simulink model "Projectsim"  (R2024a)
settings: Solver=VariableStepAuto  StartTime=0.0  StopTime=10.0  RelTol=1e-3
libraries: spsDiodeLib x8, spsCurrentMeasurementLib x4, spsGtoLib x4, spsSeriesRLCBranchLib x4, spsVoltageMeasurementLib x4, spsDCVoltageSourceLib x1, spsLinearTransformerLib x1, sps_lib x1
settings Model: Creator=yashp  LastModifiedBy=yashp

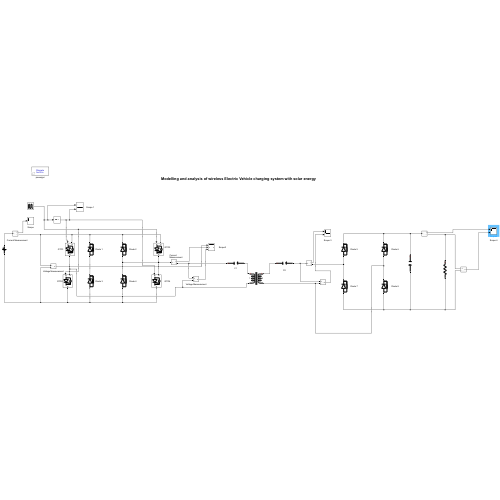
[thumbnail: Simulink's stored preview of the top-level diagram]
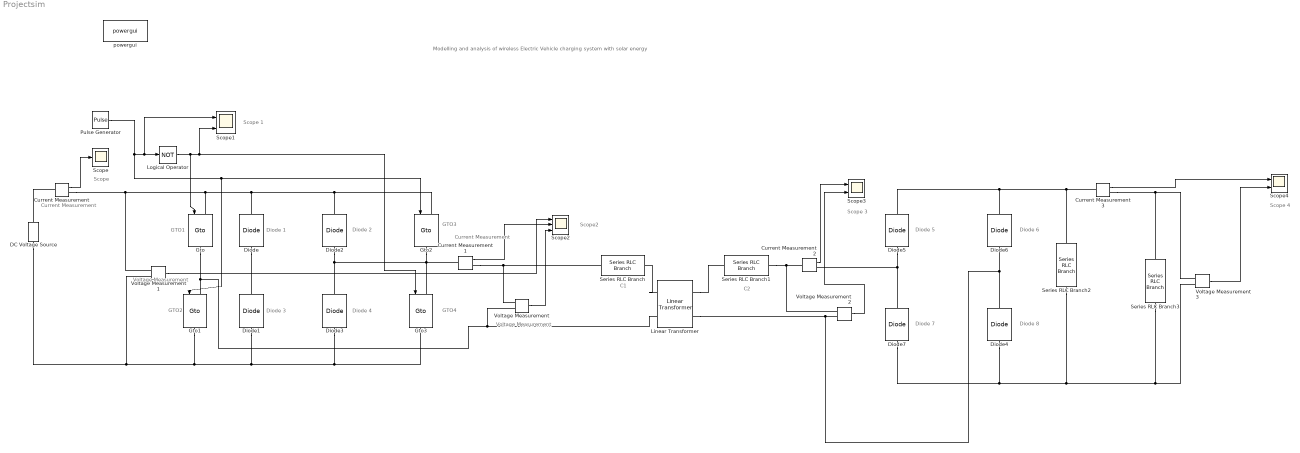
== system Projectsim ==
  note: Diode 8
  note: Diode 7
  note: Diode 6
  note: Diode 5
  note: C2
  note: C1
  note: Scope 4
  note: Scope 3
  note: Scope2
  note: Voltage Measurement
  note: Current
      | Measurement
  note: Scope 1
  note: Scope
  note: Voltage Measurement
  note: Current Measurement
  note: Diode 4
  note: Diode 3
  note: Diode 2
  note: Diode 1
  note: GTO4
  note: GTO3
  note: GTO2
  note: GTO1
  note: Modelling and analysis of wireless Electric Vehicle charging system with solar energy
  Current Measurement{,1..3} (4 alike) : spsCurrentMeasurementLib/Current Measurement  PhasorSimulation=off  OutputType=Complex  PSBequivalent=0
  DC Voltage Source : spsDCVoltageSourceLib/DC Voltage Source  Amplitude=228  Measurements=None
  Diode{,1..7} (8 alike) : spsDiodeLib/Diode  Ron=0.001  Lon=0  Vf=0.8  IC=0  UseSnubber=0  Rs=500  Cs=250e-9  Measurements=off
  Gto{,1..3} (4 alike) : spsGtoLib/Gto  Ron=0.001  Lon=0  Vf=1  Tf=10e-6  Tt=20e-6  IC=0  Rs=1e5  Cs=inf  Measurements=off
      settings: LibrarySourceBlock=sps_lib/Power Electronics/Gto
  Linear Transformer : spsLinearTransformerLib/Linear Transformer  UNITS=pu  NominalPower=[ 250e6 60 ]  winding1="[ 735e3  0.002  0.08 ]"  winding2="[ 315e3  0.002  0.08 ]"  ThreeWindings=off  winding3=[ 315e3 0.002 0.08 ]  RmLm=[ 500 500 ]  Measurements=None  DataType=off
  Logical Operator : Logic  Operator=NOT  AllPortsSameDT=off  OutDataTypeStr=boolean
  Pulse Generator : DiscretePulseGenerator  PulseType=Time based  Period=2.4096e-05  PulseWidth=50
  Scope : Scope
  Scope1 : Scope  NumInputPorts=2
  Scope2 : Scope  NumInputPorts=3
  Scope3 : Scope  NumInputPorts=2
  Scope4 : Scope  NumInputPorts=2
  Series RLC Branch : spsSeriesRLCBranchLib/Series RLC Branch  LConnTagsString=__new0  RConnTagsString=__new0  BranchType=C  Resistance=1  Inductance=1e-3  SetiL0=off  InitialCurrent=0  Capacitance=1e-6  Setx0=off  InitialVoltage=0  Measurements=None
  Series RLC Branch1 : spsSeriesRLCBranchLib/Series RLC Branch  LConnTagsString=__new0  RConnTagsString=__new0  BranchType=C  Resistance=1  Inductance=1e-3  SetiL0=off  InitialCurrent=0  Capacitance=1e-6  Setx0=off  InitialVoltage=0  Measurements=None
  Series RLC Branch2 : spsSeriesRLCBranchLib/Series RLC Branch  LConnTagsString=__new0  RConnTagsString=__new0  BranchType=C  Resistance=1  Inductance=1e-3  SetiL0=off  InitialCurrent=0  Capacitance=1e-6  Setx0=off  InitialVoltage=0  Measurements=None
  Series RLC Branch3 : spsSeriesRLCBranchLib/Series RLC Branch  LConnTagsString=__new0  RConnTagsString=__new0  BranchType=R  Resistance=100  Inductance=1e-3  SetiL0=off  InitialCurrent=0  Capacitance=1e-6  Setx0=off  InitialVoltage=0  Measurements=None
  Voltage Measurement{,1..3} (4 alike) : spsVoltageMeasurementLib/Voltage Measurement  PhasorSimulation=off  OutputType=Complex  PSBequivalent=0
  powergui : sps_lib/powergui  Priority=1  SimulationMode=Discrete  SampleTime=5e-05  frequency=60  Iterations=50  frequencyindice=0  Pbase=100e6  ErrMax=1e-4  UnitsV=kV  UnitsW=MW  buscounter=0  FunctionMessages=off  echomessages=off  EnableUseOfTLC=off  CurrentSourceSwitches=off  DisableSnubberDevices=off  DisableRonSwitches=off  DisableVfSwitches=off  DisplayEquations=off  AutomaticDiscreteSolvers=off  SolverType=Tustin/Backward Euler (TBE)  Interpol=off  ExternalGateDelay=off  methode=off  Ts=100  x0status=blocks  SPID=on  SwTol=0  HookPort=off  NonlinearTolerance=1e-4  nMaxIteration=100  ContinueOnMaxIteration=off  RestoreLinks=warning  ResistiveCurrentMeasurement=off  Frange=[0:2:500]  Ylog=off  Xlog=on  ShowGrid=off  save=off  variable=ZData  structure=0  ZoomFFT=off  StartTime=0.0  cycles=1  DisplayStyle=1  fundamental=60  FreqAxis=off  MaxFrequency=1000  frequencyindicesteady=1  RmsSteady=1  display=off
  wires:
  Current Measurement/1 -> Scope/1
  Pulse Generator/1 -> Gto1/1, Gto2/1, Scope1/1, Logical Operator/1
  Logical Operator/1 -> Scope1/2, Gto3/1, Gto/1
  Voltage Measurement1/1 -> Scope2/1
  Current Measurement1/1 -> Scope2/2
  Voltage Measurement/1 -> Scope2/3
  Current Measurement2/1 -> Scope3/1
  Voltage Measurement2/1 -> Scope3/2
  Current Measurement3/1 -> Scope4/1
  Voltage Measurement3/1 -> Scope4/2
  connections:
  DC Voltage Source/RConn1 -- Current Measurement/LConn1
  Current Measurement/RConn1 -- Voltage Measurement1/LConn1 -- Gto/LConn1 -- Diode/RConn1 -- Diode2/RConn1 -- Gto2/LConn1
  Gto/RConn1 -- Voltage Measurement/LConn2 -- Linear Transformer/LConn2 -- Gto1/LConn1
  Diode/LConn1 -- Diode1/RConn1
  Gto2/RConn1 -- Current Measurement1/LConn1 -- Diode3/RConn1 -- Diode2/LConn1 -- Gto3/LConn1
  Current Measurement1/RConn1 -- Voltage Measurement/LConn1 -- Series RLC Branch/LConn1
  Linear Transformer/LConn1 -- Series RLC Branch/RConn1
  Linear Transformer/RConn1 -- Series RLC Branch1/LConn1
  Series RLC Branch1/RConn1 -- Voltage Measurement2/LConn1 -- Current Measurement2/LConn1
  Diode5/LConn1 -- Current Measurement2/RConn1 -- Diode7/RConn1
  Diode4/RConn1 -- Linear Transformer/RConn2 -- Voltage Measurement2/LConn2 -- Diode6/LConn1
  Diode5/RConn1 -- Diode6/RConn1 -- Series RLC Branch2/LConn1 -- Current Measurement3/LConn1
  Diode7/LConn1 -- Diode4/LConn1 -- Series RLC Branch2/RConn1 -- Series RLC Branch3/RConn1 -- Voltage Measurement3/LConn2
  Current Measurement3/RConn1 -- Series RLC Branch3/LConn1 -- Voltage Measurement3/LConn1
  Voltage Measurement1/LConn2 -- DC Voltage Source/LConn1 -- Gto1/RConn1 -- Diode1/LConn1 -- Diode3/LConn1 -- Gto3/RConn1
